simulink model "IM_DiyModel"  (R2023a)
settings: Solver=VariableStepAuto  StartTime=0.0  StopTime=10.0  RelTol=1e-3
undefined symbols (not defined in the file): J, k, K_T, L_m, L_s, np, R_r, R_s, Tm, V_dr, V_qr, Vmax, w
settings Model: Creator=11048  LastModifiedBy=11048

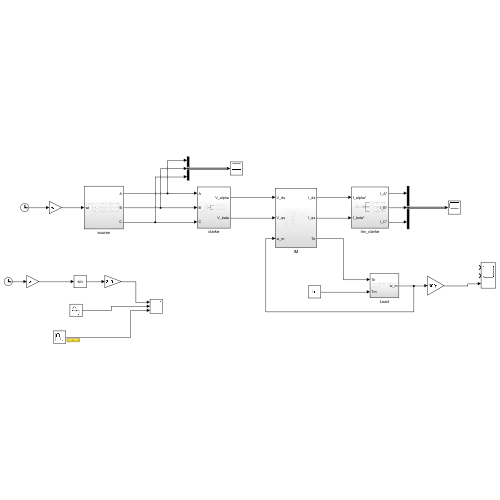
[thumbnail: Simulink's stored preview of the top-level diagram]
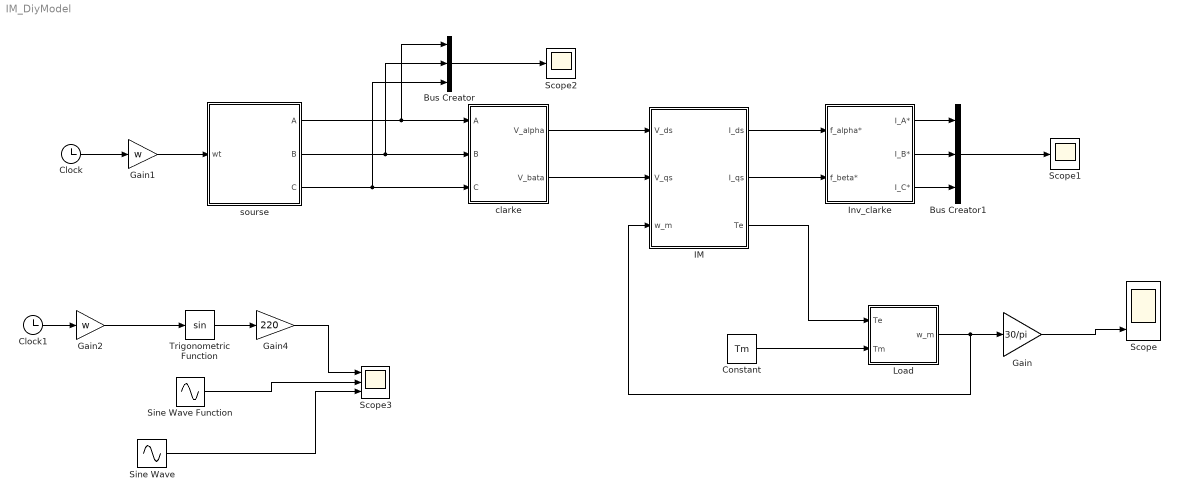
== system IM_DiyModel ==
  Bus Creator : BusCreator  Inputs=3
  Bus Creator1 : BusCreator  Inputs=3
  Clock : Clock
  Clock1 : Clock
  Constant : Constant  Value=Tm
  Gain : Gain  Gain=30/pi
  Gain1 : Gain  Gain=w
  Gain2 : Gain  Gain=w
  Gain4 : Gain  Gain=220
  IM : Subsystem
  Inv_clarke : Subsystem
  Load : Subsystem
  Scope : Scope  NumInputPorts=3
  Scope1 : Scope
  Scope2 : Scope
  Scope3 : Scope  NumInputPorts=3
  Sine Wave : Sin  Amplitude=220  Frequency=2*pi*50  SampleTime=0.00001
  Sine Wave Function : Sin  Amplitude=220  Frequency=2*pi*50  SampleTime=0.0001
  Trigonometric Function : Trigonometry
  clarke : Subsystem
  sourse : Subsystem
  wires:
  IM/3(Te) -> Load/1(Te)
  Constant/1 -> Load/2(Tm)
  Load/1(w_m) -> IM/3(w_m), Gain/1
  Gain/1 -> Scope/3
  clarke/1(V_alpha) -> IM/1(V_ds)
  clarke/2(V_bata) -> IM/2(V_qs)
  IM/2(I_qs) -> Inv_clarke/2(f_beta*)
  IM/1(I_ds) -> Inv_clarke/1(f_alpha*)
  Inv_clarke/1(I_A*) -> Bus Creator1/1
  Inv_clarke/2(I_B*) -> Bus Creator1/2
  Inv_clarke/3(I_C*) -> Bus Creator1/3
  Clock/1 -> Gain1/1
  Gain1/1 -> sourse/1(wt)
  sourse/1(A) -> Bus Creator/1, clarke/1(A)
  sourse/2(B) -> Bus Creator/2, clarke/2(B)
  sourse/3(C) -> Bus Creator/3, clarke/3(C)
  Bus Creator/1 -> Scope2/1
  Bus Creator1/1 -> Scope1/1
  Clock1/1 -> Gain2/1
  Sine Wave Function/1 -> Scope3/2
  Gain2/1 -> Trigonometric Function/1
  Trigonometric Function/1 -> Gain4/1
  Gain4/1 -> Scope3/1
  Sine Wave/1 -> Scope3/3

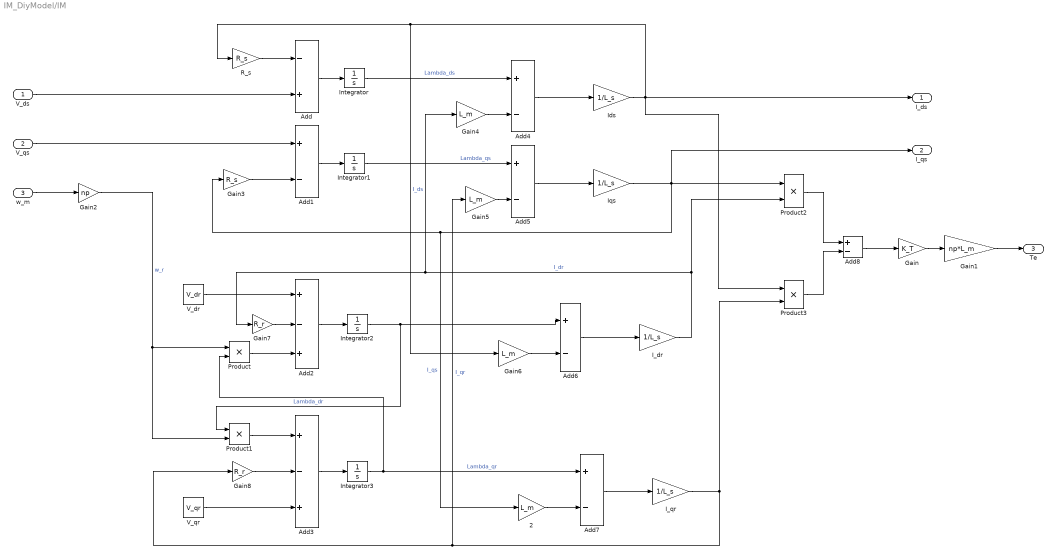
== system IM_DiyModel/IM ==
  V_ds : Inport
  V_qs : Inport  Port=2
  w_m : Inport  Port=3
  2 : Gain  Gain=L_m
  Add : Sum  Inputs=-+
  Add{1,4..8} (6 alike) : Sum  Inputs=+-
  Add2 : Sum  Inputs=+-+
  Add3 : Sum  Inputs=+-+
  Gain : Gain  Gain=K_T
  Gain1 : Gain  Gain=np*L_m
  Gain2 : Gain  Gain=np
  Gain3 : Gain  Gain=R_s
  Gain4 : Gain  Gain=L_m
  Gain5 : Gain  Gain=L_m
  Gain6 : Gain  Gain=L_m
  Gain7 : Gain  Gain=R_r
  Gain8 : Gain  Gain=R_r
  I_dr : Gain  Gain=1/L_s
  I_qr : Gain  Gain=1/L_s
  Ids : Gain  Gain=1/L_s
  Integrator{,1..3} (4 alike) : Integrator
  Iqs : Gain  Gain=1/L_s
  Product{,1..3} (4 alike) : Product
  R_s : Gain  Gain=R_s
  V_dr : Constant  Value=V_dr
  V_qr : Constant  Value=V_qr
  I_ds : Outport
  I_qs : Outport  Port=2
  Te : Outport  Port=3
  wires:
  Add5/1 -> Iqs/1
  Ids/1 -> I_ds/1, Product3/1, Gain6/1, R_s/1  "I_ds"
  Add6/1 -> I_dr/1
  Integrator2/1 -> Product1/1, Add6/1  "Lambda_dr"
  Gain3/1 -> Add1/2
  I_qr/1 -> Product3/2, Gain5/1, Gain8/1  "I_qr"
  R_s/1 -> Add/1
  Add4/1 -> Ids/1
  Product/1 -> Add2/3
  2/1 -> Add7/2
  Gain/1 -> Gain1/1
  I_dr/1 -> Product2/2, Gain4/1, Gain7/1  "I_dr"
  V_ds/1 -> Add/2
  Iqs/1 -> I_qs/1, Gain3/1, 2/1, Product2/1  "I_qs"
  Gain5/1 -> Add5/2
  Gain2/1 -> Product/1, Product1/2  "w_r"
  Product2/1 -> Add8/1
  Add/1 -> Integrator/1
  Integrator3/1 -> Add7/1, Product/2  "Lambda_qr"
  Product1/1 -> Add3/1
  V_qs/1 -> Add1/1
  V_dr/1 -> Add2/1
  Add8/1 -> Gain/1
  Integrator/1 -> Add4/1  "Lambda_ds"
  Add1/1 -> Integrator1/1
  Gain6/1 -> Add6/2
  Integrator1/1 -> Add5/1  "Lambda_qs"
  Add7/1 -> I_qr/1
  V_qr/1 -> Add3/3
  Add3/1 -> Integrator3/1
  Gain4/1 -> Add4/2
  w_m/1 -> Gain2/1
  Product3/1 -> Add8/2
  Add2/1 -> Integrator2/1
  Gain1/1 -> Te/1
  Gain7/1 -> Add2/2
  Gain8/1 -> Add3/2

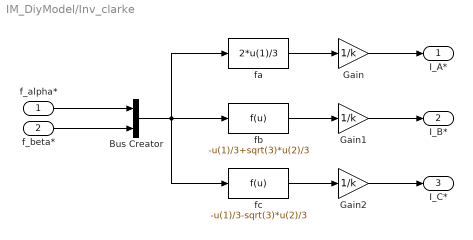
== system IM_DiyModel/Inv_clarke ==
  f_alpha* : Inport
  f_beta* : Inport  Port=2
  Bus Creator : BusCreator  Inputs=2
  Gain : Gain  Gain=1/k
  Gain1 : Gain  Gain=1/k
  Gain2 : Gain  Gain=1/k
  fa : Fcn  Expr=2*u(1)/3
  fb : Fcn  Expr=-u(1)/3+sqrt(3)*u(2)/3
  fc : Fcn  Expr=-u(1)/3-sqrt(3)*u(2)/3
  I_A* : Outport
  I_B* : Outport  Port=2
  I_C* : Outport  Port=3
  wires:
  Bus Creator/1 -> fc/1, fb/1, fa/1
  f_alpha*/1 -> Bus Creator/1
  f_beta*/1 -> Bus Creator/2
  fa/1 -> Gain/1
  Gain/1 -> I_A*/1
  fb/1 -> Gain1/1
  Gain1/1 -> I_B*/1
  fc/1 -> Gain2/1
  Gain2/1 -> I_C*/1

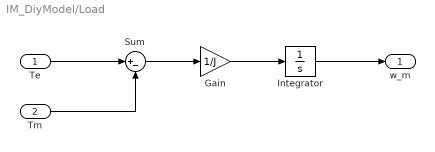
== system IM_DiyModel/Load ==
  Te : Inport
  Tm : Inport  Port=2
  Gain : Gain  Gain=1/J
  Integrator : Integrator
  Sum : Sum  Inputs=|+-
  w_m : Outport
  wires:
  Tm/1 -> Sum/2
  Integrator/1 -> w_m/1
  Sum/1 -> Gain/1
  Te/1 -> Sum/1
  Gain/1 -> Integrator/1

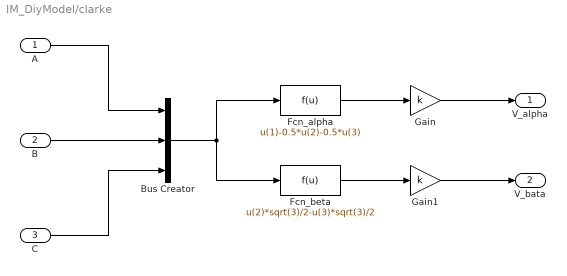
== system IM_DiyModel/clarke ==
  A : Inport
  B : Inport  Port=2
  C : Inport  Port=3
  Bus Creator : BusCreator  Inputs=3
  Fcn_alpha : Fcn  Expr=u(1)-0.5*u(2)-0.5*u(3)
  Fcn_beta : Fcn  Expr=u(2)*sqrt(3)/2-u(3)*sqrt(3)/2
  Gain : Gain  Gain=k
  Gain1 : Gain  Gain=k
  V_alpha : Outport
  V_bata : Outport  Port=2
  wires:
  Bus Creator/1 -> Fcn_beta/1, Fcn_alpha/1
  A/1 -> Bus Creator/1
  C/1 -> Bus Creator/3
  B/1 -> Bus Creator/2
  Fcn_alpha/1 -> Gain/1
  Gain/1 -> V_alpha/1
  Fcn_beta/1 -> Gain1/1
  Gain1/1 -> V_bata/1

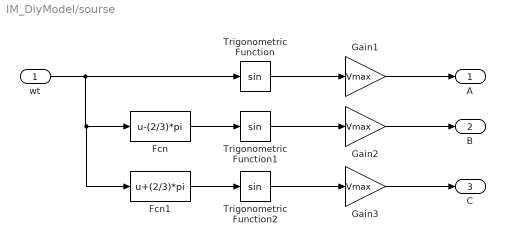
== system IM_DiyModel/sourse ==
  wt : Inport
  Fcn : Fcn  Expr=u-(2/3)*pi
  Fcn1 : Fcn  Expr=u+(2/3)*pi
  Gain1 : Gain  Gain=Vmax
  Gain2 : Gain  Gain=Vmax
  Gain3 : Gain  Gain=Vmax
  Trigonometric Function : Trigonometry
  Trigonometric Function1 : Trigonometry
  Trigonometric Function2 : Trigonometry
  A : Outport
  B : Outport  Port=2
  C : Outport  Port=3
  wires:
  Trigonometric Function/1 -> Gain1/1
  wt/1 -> Fcn1/1, Fcn/1, Trigonometric Function/1
  Fcn/1 -> Trigonometric Function1/1
  Fcn1/1 -> Trigonometric Function2/1
  Gain3/1 -> C/1
  Gain1/1 -> A/1
  Gain2/1 -> B/1
  Trigonometric Function2/1 -> Gain3/1
  Trigonometric Function1/1 -> Gain2/1
